simulink model "Sum"  (R2014a)
settings: Solver=ode1  StartTime=0.0  StopTime=10.0  RelTol=1e-3
settings Model: Creator=alunan  LastModifiedBy=anthonydelage
settings OptimizationCC: BooleanDataType=off  DefaultUnderspecifiedDataType=single  OptimizeModelRefInitCode=on  LifeSpan=1
settings HardwareCC: ProdHWDeviceType=ASIC/FPGA->ASIC/FPGA  TargetIntDivRoundTo=Floor  TargetEndianess=LittleEndian  TargetHWDeviceType=Generic->32-bit Embedded Processor  ProdEqTarget=off
settings RTWCC: SystemTargetFile=ert.tlc  TemplateMakefile=ert_default_tmf  Description=Embedded Coder  RetainRTWFile=on  ProcessScript=ert_make_rtw_hook  BuildConfiguration=Debug
settings CodeAppCC: IgnoreCustomStorageClasses=off  MATLABSourceComments=on
settings ERTTargetCC: ParMdlRefBuildCompliant=on  CompOptLevelCompliant=on  ConcurrentExecutionCompliant=on  ERTFirstTimeCompliant=on  ModelStepFunctionPrototypeControlCompliant=on  CPPClassGenCompliant=on  InlinedParameterPlacement=Hierarchical  ERTCustomFileTemplate=example_file_process.tlc  ERTFilePackagingFormat=CompactWithDataFile  ConvertIfToSwitch=on

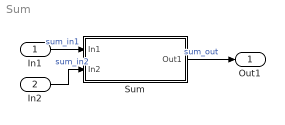
== system Sum ==
  In1 : Inport
  In2 : Inport  Port=2
  Sum : Subsystem
  Out1 : Outport
  wires:
  In1/1 -> Sum/1(In1)  "sum_in1"
  In2/1 -> Sum/2(In2)  "sum_in2"
  Sum/1(Out1) -> Out1/1  "sum_out"

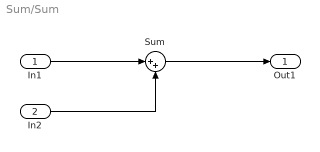
== system Sum/Sum ==
  In1 : Inport
  In2 : Inport  Port=2
  Sum : Sum  Inputs=|++
  Out1 : Outport
  wires:
  In1/1 -> Sum/1
  In2/1 -> Sum/2
  Sum/1 -> Out1/1
